simulink model "new"  (R2020a)
settings: Solver=VariableStepAuto  StartTime=0.0  StopTime=10.0  RelTol=1e-3
values from neighbouring files (symbols this model uses):
  Als_mode : value not decoded    [ALS_Project_dd.sldd]
  Carangle = 25.0    [ALS_Project_dd.sldd]    (also in Car_Angle.m = Simulink.Parameter)
  Ignition : value not decoded    [ALS_Project_dd.sldd]
  Lights : value not decoded    [ALS_Project_dd.sldd]
  Time = 2.0    [ALS_Project_dd.sldd]    (also in Car_Angle.m = Simulink.Parameter)
  Visual : value not decoded    [ALS_Project_dd.sldd]
  Weather : value not decoded    [ALS_Project_dd.sldd]
libraries: simulink x22
settings Model: Creator=hp  LastModifiedBy=hp

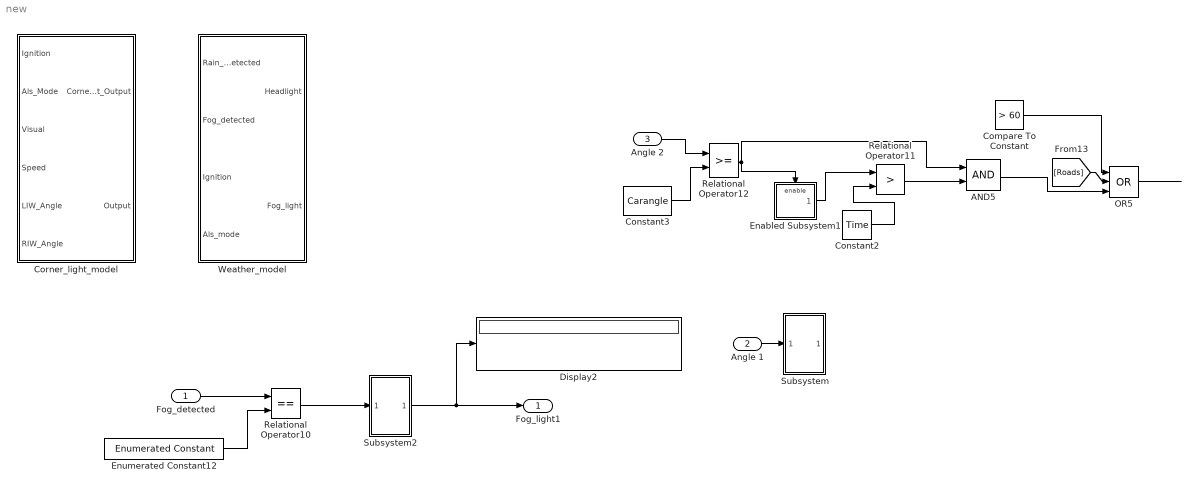
== system new ==
  Fog_detected : Inport
  Angle 1 : Inport  Port=2
  Angle 2 : Inport  Port=3
  AND5 : Logic  AllPortsSameDT=off  OutDataTypeStr=boolean
  Compare To Constant : simulink/Logic and Bit Operations/Compare To Constant  relop=>  const=60  OutDataTypeStr=boolean
  Constant2 : Constant  Value=Time
  Constant3 : Constant  Value=Carangle
  Corner_light_model : Subsystem  TreatAsAtomicUnit=on
  Display2 : Display
  Enabled Subsystem1 : Subsystem  TreatAsAtomicUnit=on
  Enumerated Constant12 : simulink/Sources/Enumerated Constant  OutDataTypeStr=Enum: Weather  Value=Weather.Fog_detected  SampleTime=inf
  OR5 : Logic  Operator=OR  Inputs=3  AllPortsSameDT=off  OutDataTypeStr=boolean
  Relational Operator10 : RelationalOperator  Operator===  OutDataTypeStr=boolean  RndMeth=Simplest
  Relational Operator11 : RelationalOperator  Operator=>  OutDataTypeStr=boolean  RndMeth=Simplest
  Relational Operator12 : RelationalOperator  OutDataTypeStr=boolean  RndMeth=Simplest
  Subsystem : Subsystem
  Subsystem2 : Subsystem
  Weather_model : Subsystem
  Fog_light1 : Outport
  wires:
  Fog_detected/1 -> Relational Operator10/1
  Enumerated Constant12/1 -> Relational Operator10/2
  Subsystem2/1(Out1) -> Display2/1, Fog_light1/1
  Relational Operator10/1 -> Subsystem2/1(In1)
  Angle 1/1 -> Subsystem/1(In1)
  [Roads] -> OR5/2
  Relational Operator11/1 -> AND5/2
  Constant3/1 -> Relational Operator12/2
  Enabled Subsystem1/1(Output) -> Relational Operator11/1
  Relational Operator12/1 -> Enabled Subsystem1/Enable, AND5/1
  AND5/1 -> OR5/3
  Constant2/1 -> Relational Operator11/2
  Compare To Constant/1 -> OR5/1
  OR5/1 -> ?
  Angle 2/1 -> Relational Operator12/1

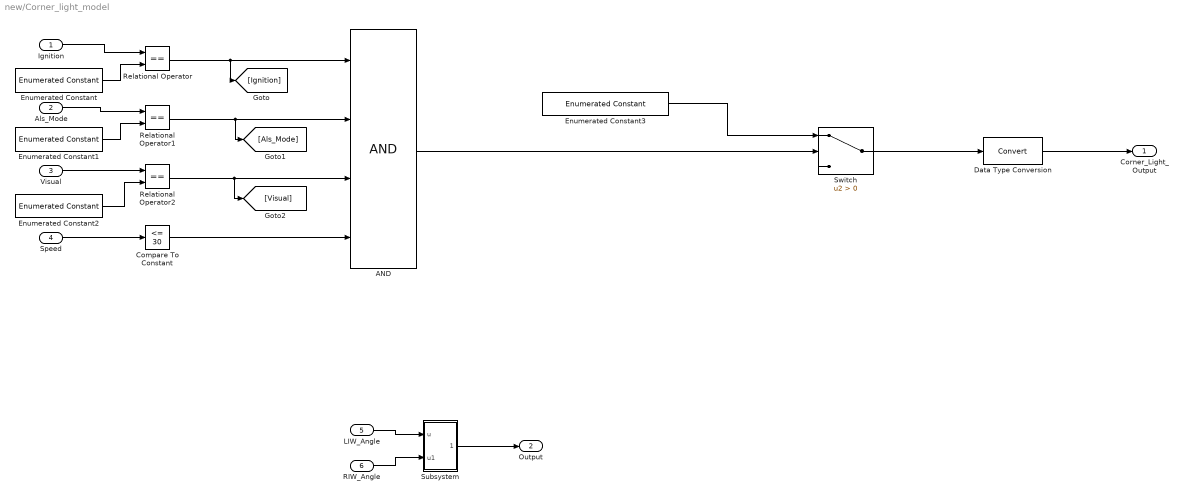
== system new/Corner_light_model ==
  Ignition : Inport
  Als_Mode : Inport  Port=2
  Visual : Inport  Port=3
  Speed : Inport  Port=4
  LIW_Angle : Inport  Port=5
  RIW_Angle : Inport  Port=6
  AND : Logic  Inputs=4  AllPortsSameDT=off  OutDataTypeStr=boolean
  Compare To Constant : simulink/Logic and Bit Operations/Compare To Constant  relop=<=  const=30  OutDataTypeStr=boolean
  Data Type Conversion : DataTypeConversion  SaturateOnIntegerOverflow=on  LockScale=on
  Enumerated Constant : simulink/Sources/Enumerated Constant  OutDataTypeStr=Enum:Ignition  Value=Ignition.On  SampleTime=inf
  Enumerated Constant1 : simulink/Sources/Enumerated Constant  OutDataTypeStr=Enum: Als_mode  Value=Als_mode.enable  SampleTime=inf
  Enumerated Constant2 : simulink/Sources/Enumerated Constant  OutDataTypeStr=Enum:Visual  Value=Visual.Night_mode  SampleTime=inf
  Enumerated Constant3 : simulink/Sources/Enumerated Constant  OutDataTypeStr=Enum: Lights  Value=Lights.Corner_Light_On  SampleTime=inf
  Relational Operator : RelationalOperator  Operator===  OutDataTypeStr=boolean  RndMeth=Simplest
  Relational Operator1 : RelationalOperator  Operator===  OutDataTypeStr=boolean  RndMeth=Simplest
  Relational Operator2 : RelationalOperator  Operator===  OutDataTypeStr=boolean  RndMeth=Simplest
  Subsystem : Subsystem
  Switch : Switch  Criteria=u2 > Threshold
  Corner_Light_Output : Outport
  Output : Outport  Port=2
  wires:
  Enumerated Constant1/1 -> Relational Operator1/2
  Visual/1 -> Relational Operator2/1
  Relational Operator2/1 -> [Visual], AND/3
  Data Type Conversion/1 -> Corner_Light_Output/1
  Ignition/1 -> Relational Operator/1
  Enumerated Constant3/1 -> Switch/1
  AND/1 -> Switch/2
  Relational Operator/1 -> [Ignition], AND/1
  Switch/1 -> Data Type Conversion/1
  Speed/1 -> Compare To Constant/1
  Als_Mode/1 -> Relational Operator1/1
  Relational Operator1/1 -> [Als_Mode], AND/2
  Enumerated Constant/1 -> Relational Operator/2
  Enumerated Constant2/1 -> Relational Operator2/2
  Compare To Constant/1 -> AND/4
  LIW_Angle/1 -> Subsystem/1(u)
  RIW_Angle/1 -> Subsystem/2(u1)
  Subsystem/1(Out1) -> Output/1

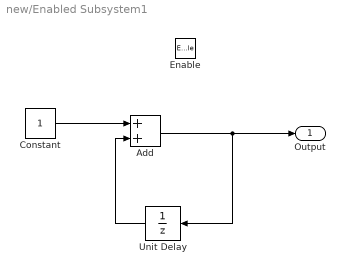
== system new/Enabled Subsystem1 ==
  Enable : EnablePort  StatesWhenEnabling=reset
  Add : Sum
  Constant : Constant
  Unit Delay : UnitDelay  SampleTime=-1  HasFrameUpgradeWarning=on
  Output : Outport  OutputWhenDisabled=reset  InitialOutput=[0]
  wires:
  Constant/1 -> Add/1
  Add/1 -> Unit Delay/1, Output/1
  Unit Delay/1 -> Add/2

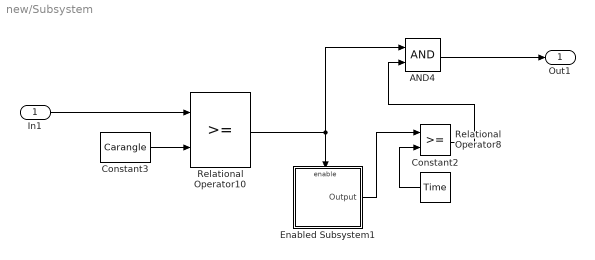
== system new/Subsystem ==
  In1 : Inport
  AND4 : Logic  AllPortsSameDT=off  OutDataTypeStr=boolean
  Constant2 : Constant  Value=Time
  Constant3 : Constant  Value=Carangle
  Enabled Subsystem1 : Subsystem  TreatAsAtomicUnit=on
  Relational Operator10 : RelationalOperator  OutDataTypeStr=boolean  RndMeth=Simplest
  Relational Operator8 : RelationalOperator  OutDataTypeStr=boolean  RndMeth=Simplest
  Out1 : Outport
  wires:
  In1/1 -> Relational Operator10/1
  Constant3/1 -> Relational Operator10/2
  Enabled Subsystem1/1(Output) -> Relational Operator8/1
  Constant2/1 -> Relational Operator8/2
  Relational Operator8/1 -> AND4/2
  Relational Operator10/1 -> AND4/1, Enabled Subsystem1/Enable
  AND4/1 -> Out1/1

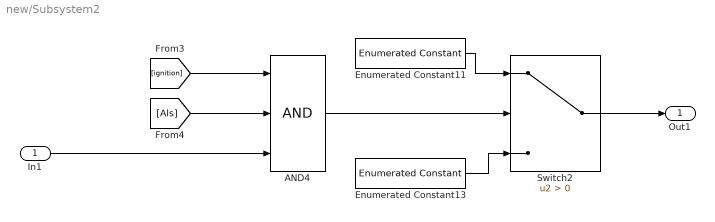
== system new/Subsystem2 ==
  In1 : Inport
  AND4 : Logic  Inputs=3  AllPortsSameDT=off  OutDataTypeStr=boolean
  Enumerated Constant11 : simulink/Sources/Enumerated Constant  OutDataTypeStr=Enum:Lights  Value=Lights.Fog_light_On  SampleTime=inf
  Enumerated Constant13 : simulink/Sources/Enumerated Constant  OutDataTypeStr=Enum:Lights  Value=Lights.Fog_light_Off  SampleTime=inf
  Switch2 : Switch  Criteria=u2 > Threshold
  Out1 : Outport
  wires:
  AND4/1 -> Switch2/2
  Switch2/1 -> Out1/1
  Enumerated Constant13/1 -> Switch2/3
  Enumerated Constant11/1 -> Switch2/1
  [Als] -> AND4/2
  [ignition] -> AND4/1
  In1/1 -> AND4/3

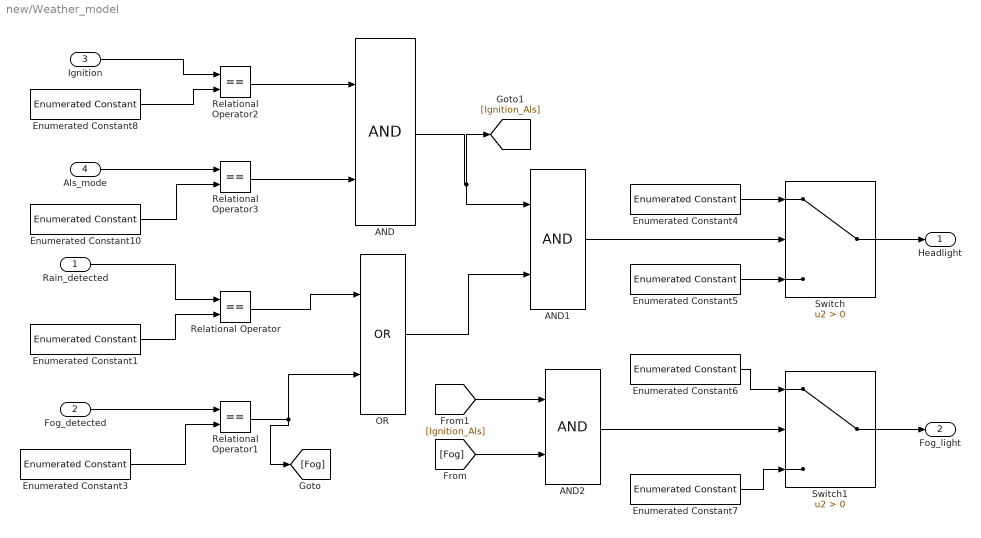
== system new/Weather_model ==
  Rain_detected : Inport
  Fog_detected : Inport  Port=2
  Ignition : Inport  Port=3
  Als_mode : Inport  Port=4
  AND : Logic  AllPortsSameDT=off  OutDataTypeStr=boolean
  AND1 : Logic  AllPortsSameDT=off  OutDataTypeStr=boolean
  AND2 : Logic  AllPortsSameDT=off  OutDataTypeStr=boolean
  Enumerated Constant1 : simulink/Sources/Enumerated Constant  OutDataTypeStr=Enum:Weather  Value=Weather.Rain_detected  SampleTime=inf
  Enumerated Constant10 : simulink/Sources/Enumerated Constant  OutDataTypeStr=Enum: Als_mode  Value=Als_mode.enable  SampleTime=inf
  Enumerated Constant3 : simulink/Sources/Enumerated Constant  OutDataTypeStr=Enum:Weather  Value=Weather.Fog_detected  SampleTime=inf
  Enumerated Constant4 : simulink/Sources/Enumerated Constant  OutDataTypeStr=Enum:Lights  Value=Lights.Low_Beam  SampleTime=inf
  Enumerated Constant5 : simulink/Sources/Enumerated Constant  OutDataTypeStr=Enum: Lights  Value=Lights.Headlights_Off  SampleTime=inf
  Enumerated Constant6 : simulink/Sources/Enumerated Constant  OutDataTypeStr=Enum:Lights  Value=Lights.Fog_light_On  SampleTime=inf
  Enumerated Constant7 : simulink/Sources/Enumerated Constant  OutDataTypeStr=Enum:Lights  Value=Lights.Fog_light_Off  SampleTime=inf
  Enumerated Constant8 : simulink/Sources/Enumerated Constant  OutDataTypeStr=Enum:Ignition  Value=Ignition.On  SampleTime=inf
  OR : Logic  Operator=OR  AllPortsSameDT=off  OutDataTypeStr=boolean
  Relational Operator{,1..3} (4 alike) : RelationalOperator  Operator===  OutDataTypeStr=boolean  RndMeth=Simplest
  Switch : Switch  Criteria=u2 > Threshold
  Switch1 : Switch  Criteria=u2 > Threshold
  Headlight : Outport
  Fog_light : Outport  Port=2
  wires:
  Enumerated Constant1/1 -> Relational Operator/2
  Enumerated Constant7/1 -> Switch1/3
  Enumerated Constant3/1 -> Relational Operator1/2
  Fog_detected/1 -> Relational Operator1/1
  Enumerated Constant5/1 -> Switch/3
  Enumerated Constant6/1 -> Switch1/1
  Relational Operator1/1 -> [Fog], OR/2
  Switch1/1 -> Fog_light/1
  Rain_detected/1 -> Relational Operator/1
  Switch/1 -> Headlight/1
  Relational Operator/1 -> OR/1
  Ignition/1 -> Relational Operator2/1
  Enumerated Constant8/1 -> Relational Operator2/2
  Enumerated Constant10/1 -> Relational Operator3/2
  Relational Operator2/1 -> AND/1
  Relational Operator3/1 -> AND/2
  AND/1 -> AND1/1, [Ignition_Als]
  OR/1 -> AND1/2
  AND1/1 -> Switch/2
  Als_mode/1 -> Relational Operator3/1
  AND2/1 -> Switch1/2
  [Fog] -> AND2/2
  [Ignition_Als] -> AND2/1
  Enumerated Constant4/1 -> Switch/1

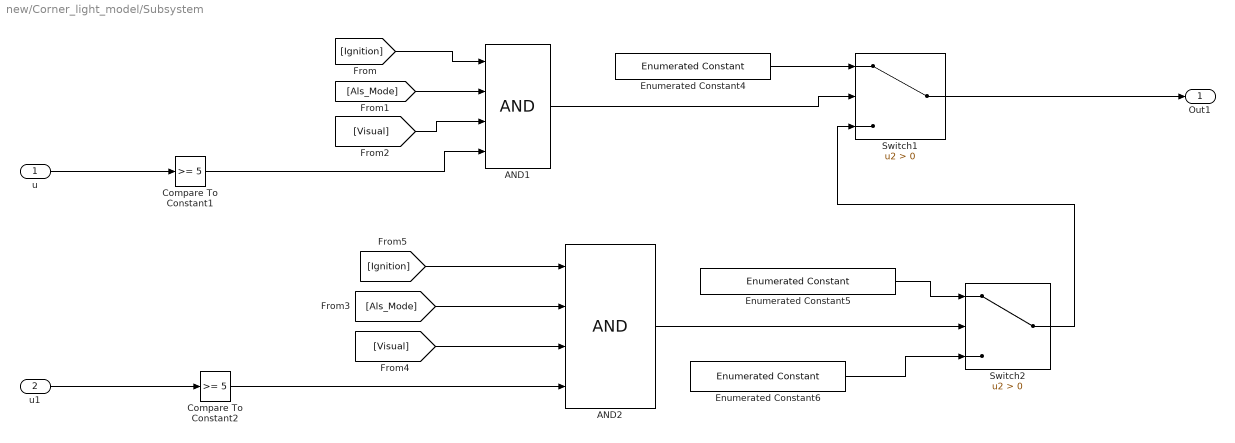
== system new/Corner_light_model/Subsystem ==
  u : Inport
  u1 : Inport  Port=2
  AND1 : Logic  Inputs=4  AllPortsSameDT=off  OutDataTypeStr=boolean
  AND2 : Logic  Inputs=4  AllPortsSameDT=off  OutDataTypeStr=boolean
  Compare To Constant1 : simulink/Logic and Bit Operations/Compare To Constant  relop=>=  const=5  OutDataTypeStr=boolean
  Compare To Constant2 : simulink/Logic and Bit Operations/Compare To Constant  relop=>=  const=5  OutDataTypeStr=boolean
  Enumerated Constant4 : simulink/Sources/Enumerated Constant  OutDataTypeStr=Enum: Lights  Value=Lights.Left_Corner_Light_On  SampleTime=inf
  Enumerated Constant5 : simulink/Sources/Enumerated Constant  OutDataTypeStr=Enum: Lights  Value=Lights.Right_Corner_Light_On  SampleTime=inf
  Enumerated Constant6 : simulink/Sources/Enumerated Constant  OutDataTypeStr=Enum: Lights  Value=Lights.Corner_Light_Off  SampleTime=inf
  Switch1 : Switch  Criteria=u2 > Threshold
  Switch2 : Switch  Criteria=u2 > Threshold
  Out1 : Outport
  wires:
  Switch2/1 -> Switch1/3
  [Visual] -> AND1/3
  Compare To Constant1/1 -> AND1/4
  Enumerated Constant5/1 -> Switch2/1
  [Ignition] -> AND1/1
  Enumerated Constant6/1 -> Switch2/3
  Compare To Constant2/1 -> AND2/4
  Enumerated Constant4/1 -> Switch1/1
  AND2/1 -> Switch2/2
  [Als_Mode] -> AND2/2
  Switch1/1 -> Out1/1
  u/1 -> Compare To Constant1/1
  [Ignition] -> AND2/1
  [Visual] -> AND2/3
  AND1/1 -> Switch1/2
  [Als_Mode] -> AND1/2
  u1/1 -> Compare To Constant2/1

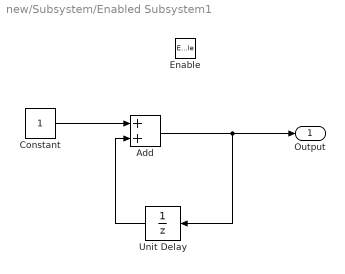
== system new/Subsystem/Enabled Subsystem1 ==
  Enable : EnablePort  StatesWhenEnabling=reset
  Add : Sum
  Constant : Constant
  Unit Delay : UnitDelay  SampleTime=-1  HasFrameUpgradeWarning=on
  Output : Outport  OutputWhenDisabled=reset  InitialOutput=[0]
  wires:
  Constant/1 -> Add/1
  Add/1 -> Unit Delay/1, Output/1
  Unit Delay/1 -> Add/2
